simulink model "no_clock_index_test_simulink"  (Simulink 7.8)
settings: Solver=VariableStepDiscrete  StartTime=0.0  StopTime=10.0  RelTol=1e-3
values from neighbouring files (symbols this model uses):
  in24b = uut.v_24bit    [no_clock_index_test.m]    (also in no_clock_test.m = double(uut.in_24bit))
  in71b1 = uut.v_71bit(1)    [no_clock_index_test.m]
  in71b2 = uut.v_71bit(2)    [no_clock_index_test.m]
  in71b3 = uut.v_71bit(3)    [no_clock_index_test.m]
settings Model: Creator=chuh  LastModifiedBy=chuh

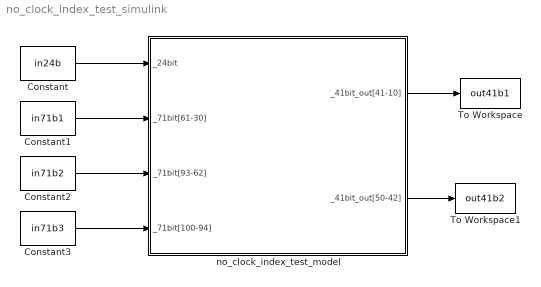
== system no_clock_index_test_simulink ==
  Constant : Constant  Value=in24b
  Constant1 : Constant  Value=in71b1
  Constant2 : Constant  Value=in71b2
  Constant3 : Constant  Value=in71b3
  To Workspace : ToWorkspace  VariableName=out41b1  SampleTime=-1  SaveFormat=Array
  To Workspace1 : ToWorkspace  VariableName=out41b2  SampleTime=-1  SaveFormat=Array
  no_clock_index_test_model : Subsystem  mask(no_clock_index_test_model){params_samples=0.001}
      mask prompts: params_samples "Sample time:"
      mask help:
      | input _24bit[31:8]
      | input _71bit[100:30]
      | output _41bit_out[50:10]
      mask Help:
      | input _24bit[31:8]
      | input _71bit[100:30]
      | output _41bit_out[50:10]
  wires:
  Constant/1 -> no_clock_index_test_model/1(_24bit)
  Constant1/1 -> no_clock_index_test_model/2(_71bit[61-30])
  Constant2/1 -> no_clock_index_test_model/3(_71bit[93-62])
  Constant3/1 -> no_clock_index_test_model/4(_71bit[100-94])
  no_clock_index_test_model/1(_41bit_out[41-10]) -> To Workspace/1
  no_clock_index_test_model/2(_41bit_out[50-42]) -> To Workspace1/1

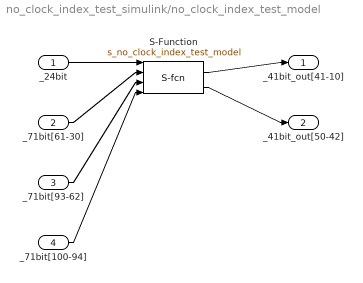
== system no_clock_index_test_simulink/no_clock_index_test_model ==
  _24bit : Inport  OutDataTypeStr=double  SampleTime=0.001
  _71bit[61-30] : Inport  Port=2  OutDataTypeStr=double  SampleTime=0.001
  _71bit[93-62] : Inport  Port=3  OutDataTypeStr=double  SampleTime=0.001
  _71bit[100-94] : Inport  Port=4  OutDataTypeStr=double  SampleTime=0.001
  S-Function : S-Function  FunctionName=s_no_clock_index_test_model  Parameters=params_samples  EnableBusSupport=off
  _41bit_out[41-10] : Outport  OutDataTypeStr=uint32  SampleTime=0.001
  _41bit_out[50-42] : Outport  Port=2  OutDataTypeStr=uint32  SampleTime=0.001
  wires:
  _24bit/1 -> S-Function/1
  _71bit[61-30]/1 -> S-Function/2
  _71bit[93-62]/1 -> S-Function/3
  _71bit[100-94]/1 -> S-Function/4
  S-Function/1 -> _41bit_out[41-10]/1
  S-Function/2 -> _41bit_out[50-42]/1
